simulink model "Half-Car"  (R2021a)
settings: Solver=VariableStepAuto  StartTime=0.0  StopTime=10.0  RelTol=1e-3
InitFcn:
  | Lf = 1.04;
  | Ksf = 33200;
  | Ksr = 43160;
  | Csf = 1760;
  | Csr = 1627;
  | Kuf =152000;
  | Cuf = 0;
  | Muf = 48;
  | Mb = 477.5;
  | Lr = 1.4;
  | Kur = 152000;
  | Cur = 0;
  | Mur = 57;
  | v=45;
  | I=1380;
libraries: pid_lib x2, simulink x1
settings Model: Creator=gandep  LastModifiedBy=vikra
settings SolverCC: AlgebraicLoopSolver=TrustRegion

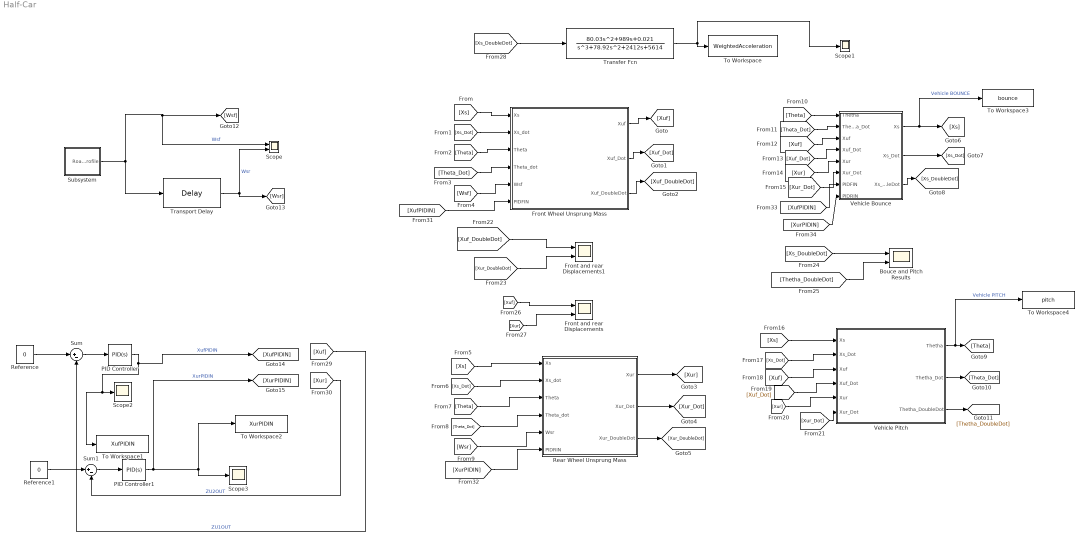
== system Half-Car ==
  Bouce and Pitch Results : Scope  NumInputPorts=2
  Front Wheel Unsprung Mass : Subsystem
  Front and rear Displacements : Scope  NumInputPorts=2
  Front and rear Displacements1 : Scope  NumInputPorts=2
  PID Controller : pid_lib/PID Controller  Controller=PID  Form=Parallel  TimeDomain=Continuous-time  UseExternalTs=off  SampleTime=-1  IntegratorMethod=Forward Euler  FilterMethod=Forward Euler  ControllerParametersSource=internal  P=0  I=100  D=0  UseFilter=on  N=100  TunerSelectOption=Transfer Function Based (PID Tuner App)  InitialConditionSource=internal  InitialConditionForIntegrator=0  InitialConditionForFilter=0  DifferentiatorICPrevScaledInput=0  ExternalReset=none  TrackingMode=off  Kt=1  LimitOutput=off  SatLimitsSource=internal  UpperSaturationLimit=inf  LowerSaturationLimit=-inf  LinearizeAsGain=on  AntiWindupMode=none  Kb=1  POutMin=[]  POutMax=[]  IOutMin=[]  IOutMax=[]  DOutMin=[]  DOutMax=[]  NOutMin=[]  NOutMax=[]  SumOutMin=[]  SumOutMax=[]  SaturationOutMin=[]  SaturationOutMax=[]  PParamMin=[]  PParamMax=[]  IParamMin=[]  IParamMax=[]  DParamMin=[]  DParamMax=[]  NParamMin=[]  NParamMax=[]  KbParamMin=[]  KbParamMax=[]  KtParamMin=[]  KtParamMax=[]  KbOutMin=[]  KbOutMax=[]  KtOutMin=[]  KtOutMax=[]  IntegratorOutMin=[]  IntegratorOutMax=[]  FilterOutMin=[]  FilterOutMax=[]  SumI1OutMin=[]  SumI1OutMax=[]  SumI2OutMin=[]  SumI2OutMax=[]  SumI3OutMin=[]  SumI3OutMax=[]  SumI4OutMin=[]  SumI4OutMax=[]  SumDOutMin=[]  SumDOutMax=[]  DifferentiatorOutMin=[]  DifferentiatorOutMax=[]  FilterDiffOutCoefMin=[]  FilterDiffOutCoefMax=[]  ReciprocalOutMin=[]  ReciprocalOutMax=[]  SumDenOutMin=[]  SumDenOutMax=[]  SumNumOutMin=[]  SumNumOutMax=[]  DivideOutMin=[]  DivideOutMax=[]  UdiffTsProdOutMin=[]  UdiffTsProdOutMax=[]  NTsProdOutMin=[]  NTsProdOutMax=[]  UintegralTsProdOutMin=[]  UintegralTsProdOutMax=[]  UngainTsProdOutMin=[]  UngainTsProdOutMax=[]  IntegratorContinuousStateAttributes=''  IntegratorStateMustResolveToSignalObject=off  IntegratorRTWStateStorageClass=Auto  FilterContinuousStateAttributes=''  FilterStateMustResolveToSignalObject=off  FilterRTWStateStorageClass=Auto  ParallelPVariant=InternalParameters  IdealPVariant=Disabled  IVariant=InternalParameters  DVariant=InternalParameters  IntegratorVariant=Continuous  SatVariant=Disabled  AWVariant=Passthrough  PCopyVariant=Disabled  TRVariant=Disabled  FdbkBlocksVariant=Forward  IdealPFdbkVariant=Disabled  SatFdbkVariant=Disabled  DerivativeFilterVariant=ContFilter  NVariant=InternalParameters  NCopyVariant=Disabled  FilterICVariant=InternalICsFilter  IntegratorICVariant=InternalICs  ExternalResetVariant=Disabled  TRSumVariant=Passthrough  SumFdbkVariant=Disabled  SumVariant=Sum_PID  TsampFilterVariant=InternalTs  TsampNgainVariant=Passthrough  TsampIntegralVariant=Passthrough  ExternalSaturationOutDataTypeStr=Inherit: Same as second input
  PID Controller1 : pid_lib/PID Controller  Controller=PID  Form=Parallel  TimeDomain=Continuous-time  UseExternalTs=off  SampleTime=-1  IntegratorMethod=Forward Euler  FilterMethod=Forward Euler  ControllerParametersSource=internal  P=0  I=100  D=0  UseFilter=on  N=100  TunerSelectOption=Transfer Function Based (PID Tuner App)  InitialConditionSource=internal  InitialConditionForIntegrator=0  InitialConditionForFilter=0  DifferentiatorICPrevScaledInput=0  ExternalReset=none  TrackingMode=off  Kt=1  LimitOutput=off  SatLimitsSource=internal  UpperSaturationLimit=inf  LowerSaturationLimit=-inf  LinearizeAsGain=on  AntiWindupMode=none  Kb=1  POutMin=[]  POutMax=[]  IOutMin=[]  IOutMax=[]  DOutMin=[]  DOutMax=[]  NOutMin=[]  NOutMax=[]  SumOutMin=[]  SumOutMax=[]  SaturationOutMin=[]  SaturationOutMax=[]  PParamMin=[]  PParamMax=[]  IParamMin=[]  IParamMax=[]  DParamMin=[]  DParamMax=[]  NParamMin=[]  NParamMax=[]  KbParamMin=[]  KbParamMax=[]  KtParamMin=[]  KtParamMax=[]  KbOutMin=[]  KbOutMax=[]  KtOutMin=[]  KtOutMax=[]  IntegratorOutMin=[]  IntegratorOutMax=[]  FilterOutMin=[]  FilterOutMax=[]  SumI1OutMin=[]  SumI1OutMax=[]  SumI2OutMin=[]  SumI2OutMax=[]  SumI3OutMin=[]  SumI3OutMax=[]  SumI4OutMin=[]  SumI4OutMax=[]  SumDOutMin=[]  SumDOutMax=[]  DifferentiatorOutMin=[]  DifferentiatorOutMax=[]  FilterDiffOutCoefMin=[]  FilterDiffOutCoefMax=[]  ReciprocalOutMin=[]  ReciprocalOutMax=[]  SumDenOutMin=[]  SumDenOutMax=[]  SumNumOutMin=[]  SumNumOutMax=[]  DivideOutMin=[]  DivideOutMax=[]  UdiffTsProdOutMin=[]  UdiffTsProdOutMax=[]  NTsProdOutMin=[]  NTsProdOutMax=[]  UintegralTsProdOutMin=[]  UintegralTsProdOutMax=[]  UngainTsProdOutMin=[]  UngainTsProdOutMax=[]  IntegratorContinuousStateAttributes=''  IntegratorStateMustResolveToSignalObject=off  IntegratorRTWStateStorageClass=Auto  FilterContinuousStateAttributes=''  FilterStateMustResolveToSignalObject=off  FilterRTWStateStorageClass=Auto  ParallelPVariant=InternalParameters  IdealPVariant=Disabled  IVariant=InternalParameters  DVariant=InternalParameters  IntegratorVariant=Continuous  SatVariant=Disabled  AWVariant=Passthrough  PCopyVariant=Disabled  TRVariant=Disabled  FdbkBlocksVariant=Forward  IdealPFdbkVariant=Disabled  SatFdbkVariant=Disabled  DerivativeFilterVariant=ContFilter  NVariant=InternalParameters  NCopyVariant=Disabled  FilterICVariant=InternalICsFilter  IntegratorICVariant=InternalICs  ExternalResetVariant=Disabled  TRSumVariant=Passthrough  SumFdbkVariant=Disabled  SumVariant=Sum_PID  TsampFilterVariant=InternalTs  TsampNgainVariant=Passthrough  TsampIntegralVariant=Passthrough  ExternalSaturationOutDataTypeStr=Inherit: Same as second input
  Rear Wheel Unsprung Mass : Subsystem
  Reference : Constant  Value=0
  Reference1 : Constant  Value=0
  Scope : Scope  NumInputPorts=2
  Scope1 : Scope
  Scope2 : Scope
  Scope3 : Scope
  Subsystem : Subsystem
  Sum : Sum  Inputs=|+-
  Sum1 : Sum  Inputs=|+-
  To Workspace : ToWorkspace  VariableName=WeightedAcceleration  SampleTime=-1
  To Workspace1 : ToWorkspace  VariableName=XufPIDIN  SaveFormat=Timeseries  SampleTime=-1
  To Workspace2 : ToWorkspace  VariableName=XurPIDIN  SaveFormat=Timeseries  SampleTime=-1
  To Workspace3 : ToWorkspace  VariableName=bounce  SaveFormat=Timeseries  SampleTime=-1
  To Workspace4 : ToWorkspace  VariableName=pitch  SaveFormat=Timeseries  SampleTime=-1
  Transfer Fcn : TransferFcn  Numerator=[80.03 989 0.021]  Denominator=[1 78.92 2412 5614]
  Transport Delay : TransportDelay  DelayTime=2.44/v
  Vehicle Bounce : Subsystem
  Vehicle Pitch : Subsystem
  wires:
  [Theta_Dot] -> Front Wheel Unsprung Mass/4(Theta_dot)
  [Theta] -> Front Wheel Unsprung Mass/3(Theta)
  [Xs_Dot] -> Front Wheel Unsprung Mass/2(Xs_dot)
  [Xs] -> Front Wheel Unsprung Mass/1(Xs)
  Front Wheel Unsprung Mass/1(Xuf) -> [Xuf]
  Front Wheel Unsprung Mass/2(Xuf_Dot) -> [Xuf_Dot]
  [Xs] -> Rear Wheel Unsprung Mass/1(Xs)
  [Xs_Dot] -> Rear Wheel Unsprung Mass/2(Xs_dot)
  [Theta] -> Rear Wheel Unsprung Mass/3(Theta)
  [Theta_Dot] -> Rear Wheel Unsprung Mass/4(Theta_dot)
  [Wsr] -> Rear Wheel Unsprung Mass/5(Wsr)
  Rear Wheel Unsprung Mass/1(Xur) -> [Xur]
  Rear Wheel Unsprung Mass/2(Xur_Dot) -> [Xur_Dot]
  [Xur] -> Vehicle Pitch/5(Xur)
  [Xur_Dot] -> Vehicle Pitch/6(Xur_Dot)
  [Xuf_Dot] -> Vehicle Pitch/4(Xuf_Dot)
  [Xuf] -> Vehicle Pitch/3(Xuf)
  [Xs_Dot] -> Vehicle Pitch/2(Xs_Dot)
  [Xs] -> Vehicle Pitch/1(Xs)
  Vehicle Pitch/2(Thetha_Dot) -> [Theta_Dot]
  Vehicle Pitch/1(Thetha) -> To Workspace4/1, [Theta]  "Vehicle PITCH"
  [Wsf] -> Front Wheel Unsprung Mass/5(Wsf)
  Vehicle Pitch/3(Thetha_DoubleDot) -> [Thetha_DoubleDot]
  Front Wheel Unsprung Mass/3(Xuf_DoubleDot) -> [Xuf_DoubleDot]
  Rear Wheel Unsprung Mass/3(Xur_DoubleDot) -> [Xur_DoubleDot]
  [Theta] -> Vehicle Bounce/1(Thetha)
  [Theta_Dot] -> Vehicle Bounce/2(Thetha_Dot)
  [Xuf] -> Vehicle Bounce/3(Xuf)
  [Xuf_Dot] -> Vehicle Bounce/4(Xuf_Dot)
  [Xur] -> Vehicle Bounce/5(Xur)
  [Xur_Dot] -> Vehicle Bounce/6(Xur_Dot)
  Vehicle Bounce/2(Xs_Dot) -> [Xs_Dot]
  Vehicle Bounce/3(Xs_DoubleDot) -> [Xs_DoubleDot]
  Transport Delay/1 -> [Wsr], Scope/2  "Wsr"
  Subsystem/1(Road profile) -> Transport Delay/1, Scope/1, [Wsf]  "Wsf"
  [Xs_DoubleDot] -> Bouce and Pitch Results/1
  [Xuf] -> Front and rear Displacements/1
  [Xur] -> Front and rear Displacements/2
  [Thetha_DoubleDot] -> Bouce and Pitch Results/2
  Transfer Fcn/1 -> To Workspace/1, Scope1/1
  [Xs_DoubleDot] -> Transfer Fcn/1
  [Xuf_DoubleDot] -> Front and rear Displacements1/1
  [Xur_DoubleDot] -> Front and rear Displacements1/2
  Sum/1 -> PID Controller/1
  PID Controller1/1 -> [XurPIDIN], Scope3/1, To Workspace2/1  "XurPIDIN"
  Sum1/1 -> PID Controller1/1
  [Xur] -> Sum1/2  "ZU2OUT"
  PID Controller/1 -> To Workspace1/1, Scope2/1, [XufPIDIN]  "XufPIDIN"
  Reference/1 -> Sum/1
  Reference1/1 -> Sum1/1
  [Xuf] -> Sum/2  "ZU1OUT"
  Vehicle Bounce/1(Xs) -> To Workspace3/1, [Xs]  "Vehicle BOUNCE"
  [XufPIDIN] -> Front Wheel Unsprung Mass/6(PIDFIN)
  [XurPIDIN] -> Rear Wheel Unsprung Mass/6(PIDRIN)
  [XufPIDIN] -> Vehicle Bounce/7(PIDFIN)
  [XurPIDIN] -> Vehicle Bounce/8(PIDRIN)

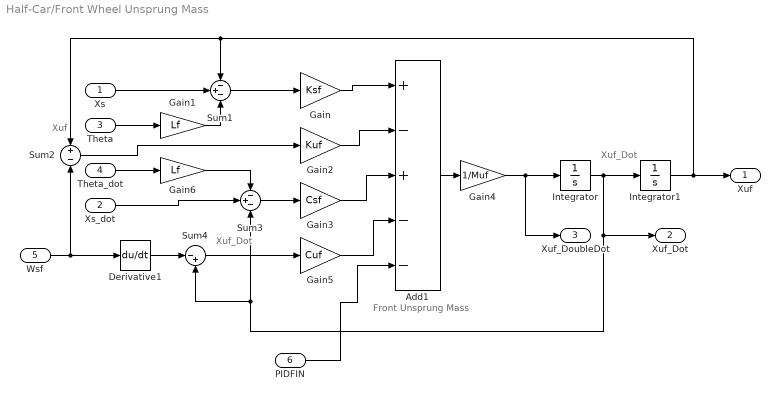
== system Half-Car/Front Wheel Unsprung Mass ==
  note: Xuf
  note: Xuf_Dot
  note: Xuf_Dot
  note: Front Unsprung Mass
  Xs : Inport
  Xs_dot : Inport  Port=2
  Theta : Inport  Port=3
  Theta_dot : Inport  Port=4
  Wsf : Inport  Port=5
  PIDFIN : Inport  Port=6
  Add1 : Sum  Inputs=+-+--
  Derivative1 : Derivative
  Gain : Gain  Gain=Ksf
  Gain1 : Gain  Gain=Lf
  Gain2 : Gain  Gain=Kuf
  Gain3 : Gain  Gain=Csf
  Gain4 : Gain  Gain=1/Muf
  Gain5 : Gain  Gain=Cuf
  Gain6 : Gain  Gain=Lf
  Integrator : Integrator
  Integrator1 : Integrator
  Sum1 : Sum  Inputs=-+-
  Sum2 : Sum  Inputs=+-
  Sum3 : Sum  Inputs=-+-
  Sum4 : Sum  Inputs=|-+
  Xuf : Outport  VectorParamsAs1DForOutWhenUnconnected=off
  Xuf_Dot : Outport  Port=2  VectorParamsAs1DForOutWhenUnconnected=off
  Xuf_DoubleDot : Outport  Port=3  VectorParamsAs1DForOutWhenUnconnected=off
  wires:
  Integrator1/1 -> Xuf/1, Sum2/1, Sum1/1
  Gain6/1 -> Sum3/1
  Integrator/1 -> Xuf_Dot/1, Sum4/2, Sum3/3, Integrator1/1
  Sum1/1 -> Gain/1
  Gain1/1 -> Sum1/3
  Xs/1 -> Sum1/2
  Theta/1 -> Gain1/1
  Add1/1 -> Gain4/1
  Gain2/1 -> Add1/2
  Gain5/1 -> Add1/4
  Theta_dot/1 -> Gain6/1
  Sum4/1 -> Gain5/1
  Derivative1/1 -> Sum4/1
  Xs_dot/1 -> Sum3/2
  Gain3/1 -> Add1/3
  Sum3/1 -> Gain3/1
  Wsf/1 -> Sum2/2, Derivative1/1
  Gain/1 -> Add1/1
  Sum2/1 -> Gain2/1
  Gain4/1 -> Xuf_DoubleDot/1, Integrator/1
  PIDFIN/1 -> Add1/5

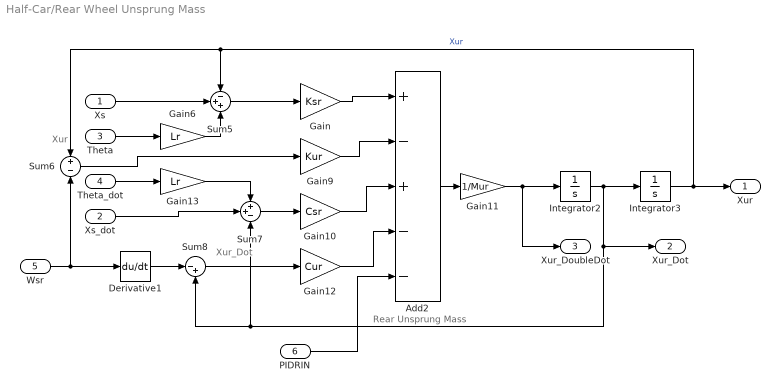
== system Half-Car/Rear Wheel Unsprung Mass ==
  note: Rear Unsprung Mass
  note: Xur_Dot
  note: Xur
  Xs : Inport
  Xs_dot : Inport  Port=2
  Theta : Inport  Port=3
  Theta_dot : Inport  Port=4
  Wsr : Inport  Port=5
  PIDRIN : Inport  Port=6
  Add2 : Sum  Inputs=+-+--
  Derivative1 : Derivative
  Gain : Gain  Gain=Ksr
  Gain10 : Gain  Gain=Csr
  Gain11 : Gain  Gain=1/Mur
  Gain12 : Gain  Gain=Cur
  Gain13 : Gain  Gain=Lr
  Gain6 : Gain  Gain=Lr
  Gain9 : Gain  Gain=Kur
  Integrator2 : Integrator
  Integrator3 : Integrator
  Sum5 : Sum  Inputs=-++
  Sum6 : Sum  Inputs=+-
  Sum7 : Sum  Inputs=++-
  Sum8 : Sum  Inputs=|-+
  Xur : Outport  VectorParamsAs1DForOutWhenUnconnected=off
  Xur_Dot : Outport  Port=2  VectorParamsAs1DForOutWhenUnconnected=off
  Xur_DoubleDot : Outport  Port=3  VectorParamsAs1DForOutWhenUnconnected=off
  wires:
  Sum6/1 -> Gain9/1
  Xs/1 -> Sum5/2
  Gain/1 -> Add2/1
  Sum5/1 -> Gain/1
  Sum8/1 -> Gain12/1
  Theta_dot/1 -> Gain13/1
  Wsr/1 -> Sum6/2, Derivative1/1
  Add2/1 -> Gain11/1
  Gain12/1 -> Add2/4
  Derivative1/1 -> Sum8/1
  Theta/1 -> Gain6/1
  Integrator3/1 -> Xur/1, Sum6/1, Sum5/1  "Xur"
  Gain13/1 -> Sum7/1
  Xs_dot/1 -> Sum7/2
  Integrator2/1 -> Xur_Dot/1, Sum7/3, Sum8/2, Integrator3/1
  Sum7/1 -> Gain10/1
  Gain6/1 -> Sum5/3
  Gain10/1 -> Add2/3
  Gain9/1 -> Add2/2
  Gain11/1 -> Xur_DoubleDot/1, Integrator2/1
  PIDRIN/1 -> Add2/5

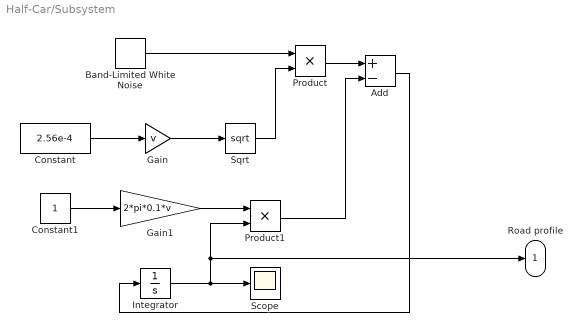
== system Half-Car/Subsystem ==
  Add : Sum  Inputs=+-
  Band-Limited White Noise : simulink/Sources/Band-Limited White Noise  Cov=[0.1]  Ts=0.01  seed=[23341]
  Constant : Constant  Value=2.56e-4
  Constant1 : Constant
  Gain : Gain  Gain=v
  Gain1 : Gain  Gain=2*pi*0.1*v
  Integrator : Integrator
  Product : Product
  Product1 : Product
  Scope : Scope
  Sqrt : Sqrt  SaturateOnIntegerOverflow=on
  Road profile : Outport  VectorParamsAs1DForOutWhenUnconnected=off
  wires:
  Gain/1 -> Sqrt/1
  Band-Limited White Noise/1 -> Product/1
  Constant/1 -> Gain/1
  Constant1/1 -> Gain1/1
  Product/1 -> Add/1
  Product1/1 -> Add/2
  Integrator/1 -> Product1/2, Road profile/1, Scope/1
  Add/1 -> Integrator/1
  Sqrt/1 -> Product/2
  Gain1/1 -> Product1/1

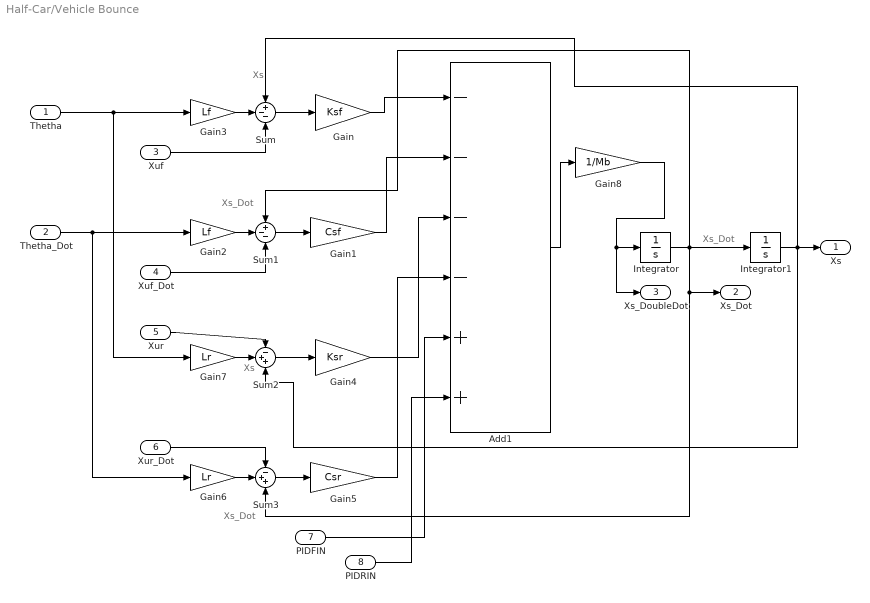
== system Half-Car/Vehicle Bounce ==
  note: Xs_Dot
  note: Xs
  note: Xs_Dot
  note: Xs
  note: Xs_Dot
  Thetha : Inport
  Thetha_Dot : Inport  Port=2
  Xuf : Inport  Port=3
  Xuf_Dot : Inport  Port=4
  Xur : Inport  Port=5
  Xur_Dot : Inport  Port=6
  PIDFIN : Inport  Port=7
  PIDRIN : Inport  Port=8
  Add1 : Sum  Inputs=----++
  Gain : Gain  Gain=Ksf
  Gain1 : Gain  Gain=Csf
  Gain2 : Gain  Gain=Lf
  Gain3 : Gain  Gain=Lf
  Gain4 : Gain  Gain=Ksr
  Gain5 : Gain  Gain=Csr
  Gain6 : Gain  Gain=Lr
  Gain7 : Gain  Gain=Lr
  Gain8 : Gain  Gain=1/Mb
  Integrator : Integrator
  Integrator1 : Integrator
  Sum : Sum  Inputs=+--
  Sum1 : Sum  Inputs=+--
  Sum2 : Sum  Inputs=-++
  Sum3 : Sum  Inputs=-++
  Xs : Outport  VectorParamsAs1DForOutWhenUnconnected=off
  Xs_Dot : Outport  Port=2  VectorParamsAs1DForOutWhenUnconnected=off
  Xs_DoubleDot : Outport  Port=3  VectorParamsAs1DForOutWhenUnconnected=off
  wires:
  Thetha_Dot/1 -> Gain2/1, Gain6/1
  Thetha/1 -> Gain7/1, Gain3/1
  Sum3/1 -> Gain5/1
  Add1/1 -> Gain8/1
  Gain3/1 -> Sum/2
  Gain2/1 -> Sum1/2
  Gain6/1 -> Sum3/2
  Xur/1 -> Sum2/1
  Gain7/1 -> Sum2/2
  Xur_Dot/1 -> Sum3/1
  Gain/1 -> Add1/1
  Gain4/1 -> Add1/3
  Integrator1/1 -> Sum2/3, Xs/1, Sum/1
  Xuf/1 -> Sum/3
  Sum1/1 -> Gain1/1
  Gain5/1 -> Add1/4
  Sum/1 -> Gain/1
  Gain1/1 -> Add1/2
  Integrator/1 -> Sum3/3, Xs_Dot/1, Integrator1/1, Sum1/1
  Gain8/1 -> Xs_DoubleDot/1, Integrator/1
  Sum2/1 -> Gain4/1
  Xuf_Dot/1 -> Sum1/3
  PIDFIN/1 -> Add1/5
  PIDRIN/1 -> Add1/6

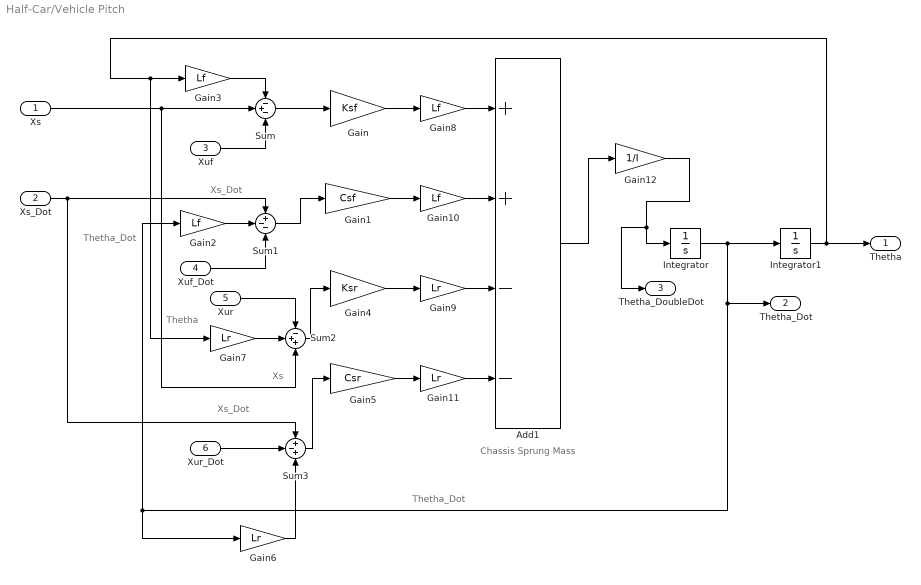
== system Half-Car/Vehicle Pitch ==
  note: Thetha_Dot
  note: Thetha
  note: Thetha_Dot
  note: Xs_Dot
  note: Chassis Sprung Mass
  note: Xs
  note: Xs_Dot
  Xs : Inport
  Xs_Dot : Inport  Port=2
  Xuf : Inport  Port=3
  Xuf_Dot : Inport  Port=4
  Xur : Inport  Port=5
  Xur_Dot : Inport  Port=6
  Add1 : Sum  Inputs=++--
  Gain : Gain  Gain=Ksf
  Gain1 : Gain  Gain=Csf
  Gain{2..3,8,10} (4 alike) : Gain  Gain=Lf
  Gain{6..7,9,11} (4 alike) : Gain  Gain=Lr
  Gain12 : Gain  Gain=1/I
  Gain4 : Gain  Gain=Ksr
  Gain5 : Gain  Gain=Csr
  Integrator : Integrator
  Integrator1 : Integrator
  Sum : Sum  Inputs=-+-
  Sum1 : Sum  Inputs=+--
  Sum2 : Sum  Inputs=-++
  Sum3 : Sum  Inputs=+-+
  Thetha : Outport  VectorParamsAs1DForOutWhenUnconnected=off
  Thetha_Dot : Outport  Port=2  VectorParamsAs1DForOutWhenUnconnected=off
  Thetha_DoubleDot : Outport  Port=3  VectorParamsAs1DForOutWhenUnconnected=off
  wires:
  Xur_Dot/1 -> Sum3/2
  Sum2/1 -> Gain4/1
  Xuf_Dot/1 -> Sum1/3
  Gain8/1 -> Add1/1
  Sum1/1 -> Gain1/1
  Integrator/1 -> Integrator1/1, Thetha_Dot/1, Gain2/1, Gain6/1
  Gain4/1 -> Gain9/1
  Gain6/1 -> Sum3/3
  Gain2/1 -> Sum1/2
  Gain1/1 -> Gain10/1
  Xur/1 -> Sum2/1
  Gain7/1 -> Sum2/2
  Gain3/1 -> Sum/1
  Gain12/1 -> Thetha_DoubleDot/1, Integrator/1
  Gain5/1 -> Gain11/1
  Add1/1 -> Gain12/1
  Xs_Dot/1 -> Sum1/1, Sum3/1
  Gain10/1 -> Add1/2
  Integrator1/1 -> Thetha/1, Gain3/1, Gain7/1
  Sum3/1 -> Gain5/1
  Sum/1 -> Gain/1
  Gain/1 -> Gain8/1
  Xuf/1 -> Sum/3
  Xs/1 -> Sum2/3, Sum/2
  Gain11/1 -> Add1/4
  Gain9/1 -> Add1/3
